simulink model "Tester"  (R2023b)
settings: Solver=VariableStepAuto  StartTime=0.0  StopTime=10.0  RelTol=1e-3
undefined symbols (not defined in the file or in its folder): canChannel
libraries: nesl_utility x9, fl_lib x8, ee_lib x6, canmsglib x3, canlib x2
settings Model: Creator=diego  LastModifiedBy=diego

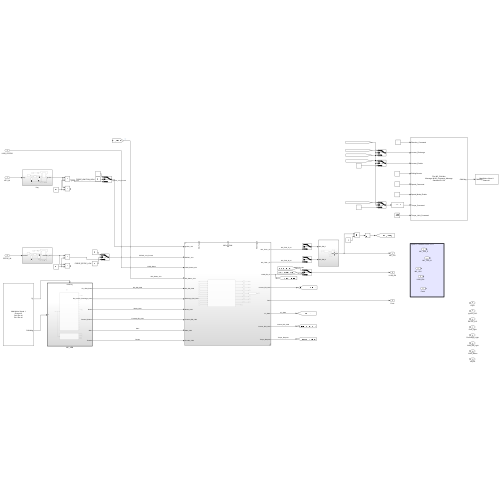
[thumbnail: Simulink's stored preview of the top-level diagram]
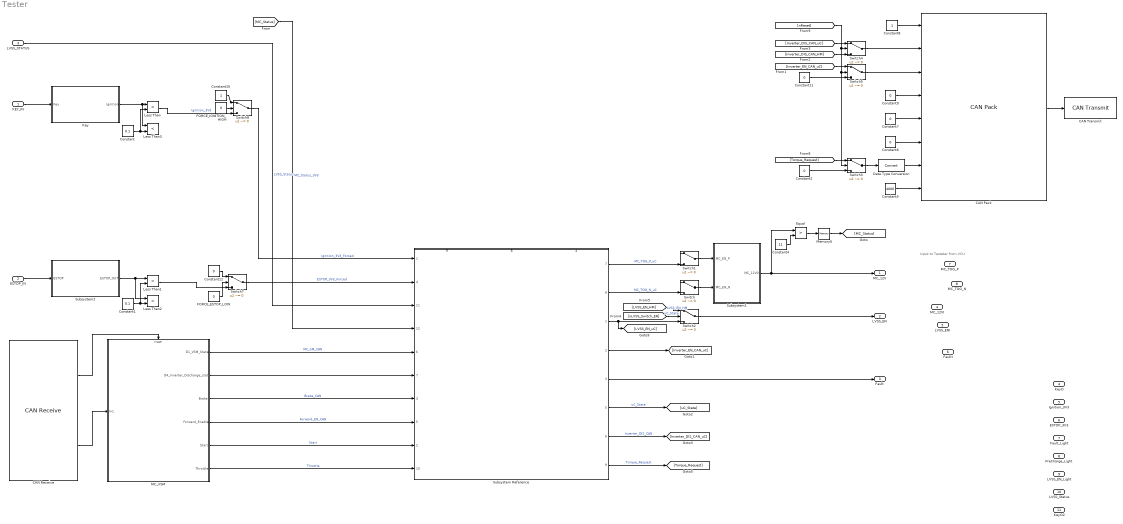
== system Tester ==
  note: Input to Testeter from VCU
  KEY_IN : Inport
  ESTOP_IN : Inport  Port=2
  LVSS_STATUS : Inport  Port=3  OutDataTypeStr=boolean
  MC_12VI : Inport  Port=4
  LVSS_ENI : Inport  Port=5
  FaultI : Inport  Port=6
  MC_TOG_P : Inport  Port=7
  MC_TOG_N : Inport  Port=8
  CAN Pack : canmsglib/CAN Pack  CANdbFile=C:\Users\heyka\MATLAB\Projects\VCU_C\MC_CAN.dbc  MsgList=M192_Command_Message  MsgName=M192_Command_Message  MsgIDType=Standard (11-bit identifier)  MsgIdentifier=192  MsgLength=8  Remote=off  ApplyMinMax=off  BusOutput=off  SignalInfo={'Direction_Command','32','1','LE','unsigned','Standard','0','1','0','0','1';'Inverter_Discharge','41','1','LE','unsigned','Standard','0','1','0','0','1';'Inverter_Enable','40','1','LE','unsigned','Standard','0','1','0','0','1';'RollingCounter','44','4','LE','unsigned','Standard','0','1','0','0','15';'Speed_Command','16','16','LE','signed','Standard','0','1','0','-32768','32767';'Speed_Mode_Enable','42','1','LE','unsigned','Standard','0','1','0','0','1';'Torque_Command','0','16','LE','signed','Standard','0','0.1','0','-3276.8','3276.7';'Torque_Limit_Command','48','16','LE','signed','Standard','0','0.1','0','-3276.8','3276.7'}
      settings: LibrarySourceBlock=canlib/CAN Pack  DataFormat=CANdb specified signals
  CAN Receive : canlib/CAN Receive  BlockHandle=405.006  Device=MathWorks Virtual 1 (Channel 2)  DeviceMenu=MathWorks Virtual 1 (Channel 2)  ObjConstructor=canChannel('MathWorks', 'Virtual 1', 2)  EnableStandardIDsFilter=off  StdIDsCombo=Allow all  StandardIDs=0  EnableExtendedIDsFilter=off  ExtIDsCombo=Allow all  ExtendedIDs=0  SampleTime=0.01  MsgsPerTimestep=all  InternalFilterUpdateStatus=on  BusOutput=off
  CAN Transmit : canlib/CAN Transmit  BlockHandle=406.006  Device=MathWorks Virtual 1 (Channel 1)  DeviceMenu=MathWorks Virtual 1 (Channel 1)  ObjConstructor=canChannel('MathWorks', 'Virtual 1', 1)  EnableEventTransmit=off  EnablePeriodicTransmit=off  MessagePeriod=1.000
  Constant : Constant  Value=0.1
  Constant1 : Constant  Value=0.1
  Constant10 : Constant  OutDataTypeStr=boolean
  Constant{2,6..7,9,11} (5 alike) : Constant  Value=0
  Constant12 : Constant  Value=0  OutDataTypeStr=boolean
  Constant4 : Constant  Value=11
  Constant5 : Constant  Value=4000
  Constant8 : Constant
  Data Type Conversion : DataTypeConversion  OutMin=[-32768]  OutMax=[32767]  SaturateOnIntegerOverflow=off  RndMeth=Floor
  Equal : RelationalOperator  Operator=>  OutDataTypeStr=boolean  RndMeth=Simplest  InputSameDT=off
  FORCE_ESTOP_LOW : Constant  Value=0
  FORCE_IGNITION_HIGH : Constant  Value=0
  Key : Subsystem
  Less Than{,1..3} (4 alike) : RelationalOperator  Operator=<  OutDataTypeStr=boolean  RndMeth=Simplest  InputSameDT=off
  MC_VSM : Subsystem  TreatAsAtomicUnit=on
  Memory6 : Memory
  Subsystem Reference : Subsystem  ReferencedSubsystem=MCuC_CAN
      settings: PortSchema="{\"entries\":[{\"content\":{\"sides\":[{\"content\":{\"connectorIds\":[\"In1\",\"In4\",\"In11\",\"In12\",\"In6\",\"In7\",\"In3\",\"In5\",\"In2\",\"In10\"]},\"type\":\"ConnectorPlacement.EquallySpacedRectSide\",\"uuid\":\"ad24675a-cf45-4ebd-8a91-6dc83f3b6f0e\"},{\"content\":{\"connectorIds\":[\"Out7\",\"Out8\",\"Out1\",\"Out2\",\"Out3\",\"Out5\",\"Out6\",\"Out9\"],\"side\":\"RIGHT\"},\"type\":\"ConnectorPlacement.EquallySpacedRectSide\",\"uuid\":\"d727ad1f-9d18-4e4b-88a0-ff4b62c4d504\"},{\"content\":{\"connectorIds\":[\"In9\",\"In8\",\"Out4\"],\"side\":\"TOP\"},\"type\":\"ConnectorPlacement.EquallySpacedRectSide\",\"uuid\":\"0dd4e640-1d3d-4994-a378-fd1340433361\"}]},\"type\":\"ConnectorPlacement.EquallySpacedConnector\",\"uuid\":\"60e23daf-f786-4411-86d8-86e23e1960b1\"}],\"packageUris\":[\"http://schema.mathworks.com/mf0/Connector/R2020b\"],\"version\":\"1.0\"}"
  Subsystem1 : Subsystem
  Subsystem2 : Subsystem
  Switch{,1..5} (6 alike) : Switch  Criteria=u2 ~= 0  SaturateOnIntegerOverflow=off  InputSameDT=off
  Switch7 : Switch  Criteria=u2 ~= 0  OutDataTypeStr=boolean  SaturateOnIntegerOverflow=off  InputSameDT=off
  Switch8 : Switch  Criteria=u2 ~= 0  OutDataTypeStr=boolean  SaturateOnIntegerOverflow=off  InputSameDT=off
  MC_12V : Outport
  LVSS_EN : Outport  Port=2
  Fault : Outport  Port=3
  KeyO : Outport  Port=4
  Ignition_3V3 : Outport  Port=5
  ESTOP_3V3 : Outport  Port=6
  Fault_Light : Outport  Port=7
  PreCharge_Light : Outport  Port=8
  LVSS_EN_Light : Outport  Port=9
  LVSS_Status : Outport  Port=10
  KeyO2 : Outport  Port=11
  wires:
  Subsystem Reference/2 -> [Inverter_EN_CAN_uC]
  Subsystem Reference/8 -> Switch/3  "MC_TOG_N_uC"
  Subsystem Reference/6 -> [Inverter_DIS_CAN_uC]  "Inverter_DIS_CAN"
  FORCE_ESTOP_LOW/1 -> Switch7/2
  Constant7/1 -> CAN Pack/5
  [Inverter_EN_CAN_uC] -> Switch5/1
  FORCE_IGNITION_HIGH/1 -> Switch8/2
  Less Than/1 -> Switch8/3  "Ignition_3V3"
  Constant10/1 -> Switch8/1
  LVSS_STATUS/1 -> Subsystem Reference/11  "LVSS_Status"
  Constant12/1 -> Switch7/1
  [Inverter_DIS_CAN_uC] -> Switch4/1
  KEY_IN/1 -> Key/1(Key)
  Subsystem Reference/9 -> [Torque_Request]  "Torque_Request"
  Switch1/1 -> Subsystem1/1(MC_EN_P)
  CAN Receive/1 -> MC_VSM/Trigger
  Switch7/1 -> Subsystem Reference/4  "ESTOP_3V3_Forced"
  Subsystem2/1(ESTOP_OUT) -> Less Than1/1, Less Than2/1
  [LVSS_EN_HM] -> Switch2/1  "LVSS_EN_HM"
  Constant2/1 -> Switch3/3
  Subsystem Reference/5 -> [uC_State]  "uC_State"
  MC_VSM/6(Throttle) -> Subsystem Reference/10  "Throttle"
  CAN Pack/1 -> CAN Transmit/1
  [MC_Status] -> Subsystem Reference/12  "MC_Status_3V3"
  CAN Receive/2 -> MC_VSM/1(In1)
  [nReset] -> Switch3/2, Switch5/2, Switch4/2
  ESTOP_IN/1 -> Subsystem2/1(ESTOP)
  MC_VSM/5(Start) -> Subsystem Reference/2  "Start"
  Subsystem Reference/7 -> Switch1/3  "MC_TOG_P_uC"
  [nLVSS_Switch_EN] -> Switch2/2  "uC_State"
  MC_VSM/2(D4_Inverter_Discharge_state) -> Subsystem Reference/7
  Switch8/1 -> Subsystem Reference/1  "Ignition_3V3_Forced"
  Subsystem Reference/1 -> [LVSS_EN_uC], Switch2/3
  Switch/1 -> Subsystem1/2(MC_EN_N)
  Constant1/1 -> Less Than1/2, Less Than2/2
  Constant11/1 -> Switch5/3
  Data Type Conversion/1 -> CAN Pack/7
  Constant6/1 -> CAN Pack/6
  Constant5/1 -> CAN Pack/8
  Equal/1 -> Memory6/1
  MC_VSM/1(D1_VSM_State) -> Subsystem Reference/6  "MC_SM_CAN"
  Constant4/1 -> Equal/2
  Key/1(Ignition) -> Less Than3/1, Less Than/1
  MC_VSM/4(Forward_Enable) -> Subsystem Reference/5  "Forward_EN_CAN"
  Switch2/1 -> LVSS_EN/1
  MC_VSM/3(Brake) -> Subsystem Reference/3  "Brake_CAN"
  [Inverter_DIS_CAN_HM] -> Switch4/3
  Switch3/1 -> Data Type Conversion/1
  Switch4/1 -> CAN Pack/2
  Constant/1 -> Less Than/2, Less Than3/2
  Subsystem1/1(MC_12V0) -> MC_12V/1, Equal/1
  Switch5/1 -> CAN Pack/3
  Less Than1/1 -> Switch7/3
  Subsystem Reference/3 -> Fault/1
  Constant8/1 -> CAN Pack/1
  Constant9/1 -> CAN Pack/4
  [Torque_Request] -> Switch3/1
  Memory6/1 -> [MC_Status]

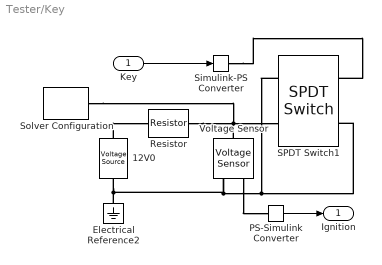
== system Tester/Key ==
  Key : Inport
  12V0 : ee_lib/Sources/Voltage Source  dc_voltage=12 V  ac_voltage=0 V  ac_shift=0 rad  ac_frequency=60 Hz  noise_mode=ee.enum.sources.noise.Disabled  PSD=0 V^2/Hz  sample_time=1e-3 s  repeatability=ee.enum.sources.repeatability.NotRepeatable  user_seed=0  auto_seed=3499211588  i_specify=off  i_priority=None  i=0 A  i_nominal_specify=off  i_nominal_unit=A  i_nominal_value=1  v_specify=off  v_priority=None  v=0 V  v_nominal_specify=off  v_nominal_unit=V  v_nominal_value=1
  Electrical Reference2 : fl_lib/Electrical/Electrical Elements/Electrical Reference
  PS-Simulink Converter : nesl_utility/PS-Simulink Converter  PhysicalDomain=network_engine_domain  SubClassName=ps_output  LeftPortType=input  RightPortType=output  PseudoPeriodic=off  Frequencies=[]  VectorFormat=inherit  Unit=inherit  AffineConversion=off
  Resistor : fl_lib/Electrical/Electrical Elements/Resistor  R=10000 Ohm  i_specify=off  i_priority=None  i=0 A  i_nominal_specify=off  i_nominal_unit=A  i_nominal_value=1  v_specify=off  v_priority=None  v=0 V  v_nominal_specify=off  v_nominal_unit=V  v_nominal_value=1
  SPDT Switch1 : ee_lib/Switches & Breakers/SPDT Switch  R_closed=0.01 Ohm  G_open=1e-10 S  Threshold=0.5 V  Width=0 V  model_dynamics=0  t_on=1e-3 s  t_off=1e-3 s  initial_vT=0 V
  Simulink-PS Converter : nesl_utility/Simulink-PS Converter  PhysicalDomain=network_engine_domain  SubClassName=ps_input  LeftPortType=input  RightPortType=output  PseudoPeriodic=off  Frequencies=[]  NoiseDistribution=none  NoiseParameters=[]  Unit=1  AffineConversion=off  FilteringAndDerivatives=provide  SimscapeFilterOrder=1  InputFilterTimeConstant=0.001  UdotUserProvided=0
  Solver Configuration : nesl_utility/Solver Configuration  PhysicalDomain=network_engine_domain  SubClassName=solver  LeftPortType=input  RightPortType=generic  Tones=[]  Harmonics=[]  SimulateNoise=off  Profile=off  UseLocalSampling=off  EnableSwitchedLinearOptims=on  FrequencyDomain=off  UseCCode=off  RelTol=0.001  AbsTol=0.001  MinStep=1e-09  ToWorkspace=off  RevertToSquareIcSolve=off  NumHomotopyIterations=100  PhasorMode=off  PhasorModeNumHarmonics=1  ConsistencySolver=NEWTON_XTOL_AFTER_FTOL  IndexReductionMethod=DerivativeReplacement  DoDC=off  ResidualTolerance=1e-09  ConsistencyTolSource=GLOBAL  ConsistencyAbsTol=0.001  ConsistencyRelTol=0.001  ConsistencyTolFactor=0.001  UseLocalSolver=off  LocalSolverChoice=NE_BACKWARD_EULER_ADVANCER  ResolveIndetEquations=on  FunctionEvalNumThread=1  LocalSolverSampleTime=0.001  DoFixedCost=off  MaxNonlinIter=3  MaxModeIter=2  ComputeImpulses=off  ImpulseIterations=2  LinearAlgebra=auto  LinearAlgebraNumThread=0  EquationFormulation=NE_TIME_EF  DelaysMemoryBudget=1024  AutomaticFiltering=on  FilteringTimeConstant=0.001  PartitionStorageMethod=AS_NEEDED  PartitionMemoryBudget=1024  PartitionMethod=ROBUST  MultibodyUseLocalSolver=off  MultibodyLocalSolverChoice=ODE1  MultibodyLocalSolverSampleTime=0.001
  Voltage Sensor : fl_lib/Electrical/Electrical Sensors/Voltage Sensor
  Ignition : Outport
  wires:
  PS-Simulink Converter/1 -> Ignition/1
  Key/1 -> Simulink-PS Converter/1
  connections:
  12V0/LConn1 -- Resistor/LConn1
  Resistor/RConn1 -- Solver Configuration/RConn1 -- Voltage Sensor/LConn1 -- SPDT Switch1/RConn2
  Electrical Reference2/LConn1 -- SPDT Switch1/RConn1 -- SPDT Switch1/LConn2 -- Voltage Sensor/RConn2 -- 12V0/RConn1
  Simulink-PS Converter/RConn1 -- SPDT Switch1/LConn1
  Voltage Sensor/RConn1 -- PS-Simulink Converter/LConn1

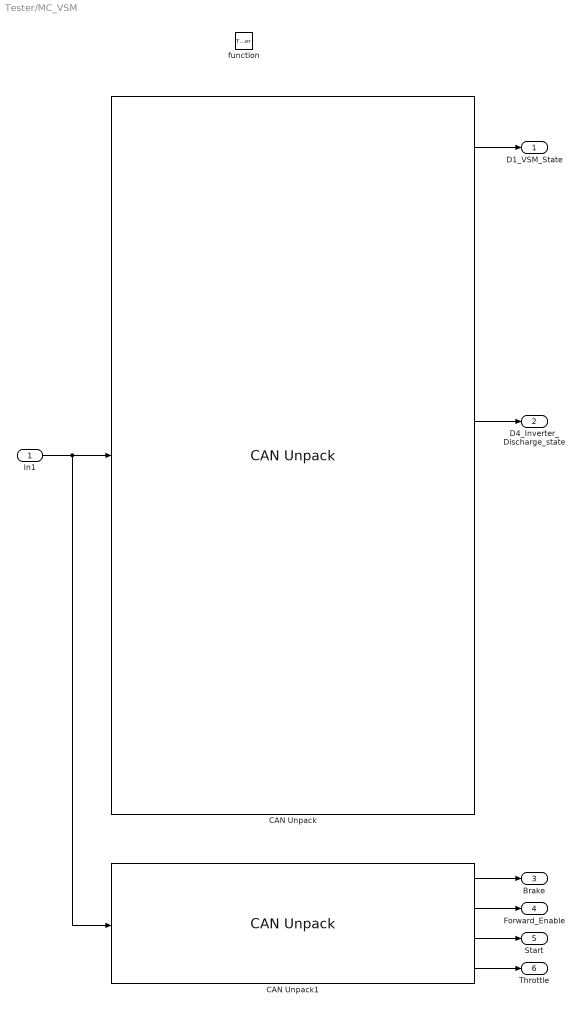
== system Tester/MC_VSM ==
  In1 : Inport
  function : TriggerPort  TriggerType=function-call  VariantControl=(inherit)
  CAN Unpack : canmsglib/CAN Unpack  CANdbFile=C:\Users\heyka\MATLAB\Projects\VCU_C\MC_CAN.dbc  MsgList=M170_Internal_States  MsgName=M170_Internal_States  MsgIDType=Standard (11-bit identifier)  MsgIdentifier=170  MsgLength=8  SignalInfo={'D1_PWM_Frequency','8','8','LE','unsigned','Standard','0','1','0','0','255';'D1_VSM_State','0','8','LE','unsigned','Standard','0','1','0','0','15';'D2_Inverter_State','16','8','LE','unsigned','Standard','0','1','0','0','255';'D3_Relay_1_Status','24','1','LE','unsigned','Standard','0','1','0','0','1';'D3_Relay_2_Status','25','1','LE','unsigned','Standard','0','1','0','0','1';'D3_Relay_3_Status','26','1','LE','unsigned','Standard','0','1','0','0','1';'D3_Relay_4_Status','27','1','LE','unsigned','Standard','0','1','0','0','1';'D3_Relay_5_Status','28','1','LE','unsigned','Standard','0','1','0','0','1';'D3_Relay_6_Status','29','1','LE','unsigned','Standard','0','1','0','0','1';'D4_Inverter_Discharge_State','37','3','LE','unsigned','Standard','0','1','0','0','7';'D4_Inverter_Run_Mode','32','1','LE','unsigned','Standard','0','1','0','0','1';'D5_Inverter_Command_Mode','40','1','LE','unsigned','Standard','0','1','0','0','1';'D5_Rolling_Counter','44','4','LE','unsigned','Standard','0','1','0','0','15';'D6_Inverter_Enable_Lockout','55','1','LE','unsigned','Standard','0','1','0','0','1';'D6_Inverter_Enable_State','48','1','LE','unsigned','Standard','0','1','0','0','1';'D6_Start_Mode_Active','54','1','LE','unsigned','Standard','0','1','0','0','1';'D7_BMS_Active','57','1','LE','unsigned','Standard','0','1','0','0','1';'D7_BMS_Torque_Limiting','58','1','LE','unsigned','Standard','0','1','0','0','1';'D7_Direction_Command','56','1','LE','unsigned','Standard','0','1','0','0','1';'D7_Low_Speed_Limiting','61','1','LE','unsigned','Standard','0','1','0','0','1';'D7_Max_Speed_Limiting','59','1','LE','unsigned','Standard','0','1','0','0','1'}  IDPort=off  TimestampPort=off  ErrorPort=off  RemotePort=off  LengthPort=off  StatusPort=off  ApplyMinMax=off
      settings: LibrarySourceBlock=canlib/CAN Unpack  DataFormat=CANdb specified signals
  CAN Unpack1 : canmsglib/CAN Unpack  CANdbFile=C:\Users\heyka\MATLAB\Projects\VCU_C\PRJDB.dbc  MsgList=N8_TPDO0  MsgName=N8_TPDO0  MsgIDType=Standard (11-bit identifier)  MsgIdentifier=392  MsgLength=5  SignalInfo={'Brake','1','16','LE','signed','Standard','0','1','0','0','494967295';'Forward_Enable','0','1','LE','unsigned','Standard','0','1','0','0','494967295';'Start','17','1','LE','unsigned','Standard','0','1','0','-Inf','Inf';'Throttle','18','16','LE','signed','Standard','0','1','0','-32768','32767'}  IDPort=off  TimestampPort=off  ErrorPort=off  RemotePort=off  LengthPort=off  StatusPort=off  ApplyMinMax=off
      settings: LibrarySourceBlock=canlib/CAN Unpack  DataFormat=CANdb specified signals
  D1_VSM_State : Outport
  D4_Inverter_Discharge_state : Outport  Port=2
  Brake : Outport  Port=3  OutDataTypeStr=int32
  Forward_Enable : Outport  Port=4  OutDataTypeStr=uint32
  Start : Outport  Port=5  OutDataTypeStr=uint32
  Throttle : Outport  Port=6  OutDataTypeStr=int32
  wires:
  In1/1 -> CAN Unpack1/1, CAN Unpack/1
  CAN Unpack/2 -> D1_VSM_State/1
  CAN Unpack/10 -> D4_Inverter_Discharge_state/1
  CAN Unpack1/1 -> Brake/1
  CAN Unpack1/2 -> Forward_Enable/1
  CAN Unpack1/3 -> Start/1
  CAN Unpack1/4 -> Throttle/1

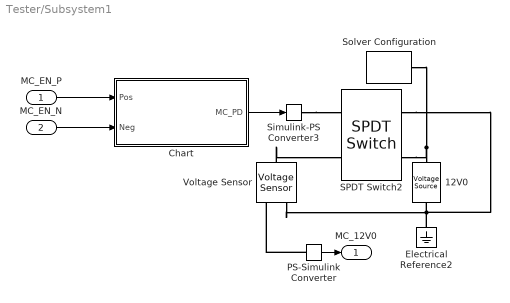
== system Tester/Subsystem1 ==
  MC_EN_P : Inport
  MC_EN_N : Inport  Port=2
  12V0 : ee_lib/Sources/Voltage Source  dc_voltage=12 V  ac_voltage=0 V  ac_shift=0 rad  ac_frequency=60 Hz  noise_mode=ee.enum.sources.noise.Disabled  PSD=0 V^2/Hz  sample_time=1e-3 s  repeatability=ee.enum.sources.repeatability.NotRepeatable  user_seed=0  auto_seed=3890346746  i_specify=off  i_priority=None  i=0 A  i_nominal_specify=off  i_nominal_unit=A  i_nominal_value=1  v_specify=off  v_priority=None  v=0 V  v_nominal_specify=off  v_nominal_unit=V  v_nominal_value=1
  Chart : Stateflow chart  TreatAsAtomicUnit=on
  Electrical Reference2 : fl_lib/Electrical/Electrical Elements/Electrical Reference
  PS-Simulink Converter : nesl_utility/PS-Simulink Converter  PhysicalDomain=network_engine_domain  SubClassName=ps_output  LeftPortType=input  RightPortType=output  PseudoPeriodic=off  Frequencies=[]  VectorFormat=inherit  Unit=inherit  AffineConversion=off
  SPDT Switch2 : ee_lib/Switches & Breakers/SPDT Switch  R_closed=0.01 Ohm  G_open=1e-6 S  Threshold=0.5 V  Width=0 V  model_dynamics=0  t_on=1e-3 s  t_off=1e-3 s  initial_vT=0 V
  Simulink-PS Converter3 : nesl_utility/Simulink-PS Converter  PhysicalDomain=network_engine_domain  SubClassName=ps_input  LeftPortType=input  RightPortType=output  PseudoPeriodic=off  Frequencies=[]  NoiseDistribution=none  NoiseParameters=[]  Unit=1  AffineConversion=off  FilteringAndDerivatives=provide  SimscapeFilterOrder=1  InputFilterTimeConstant=0.001  UdotUserProvided=0
  Solver Configuration : nesl_utility/Solver Configuration  PhysicalDomain=network_engine_domain  SubClassName=solver  LeftPortType=input  RightPortType=generic  Tones=[]  Harmonics=[]  SimulateNoise=off  Profile=off  UseLocalSampling=off  EnableSwitchedLinearOptims=on  FrequencyDomain=off  UseCCode=off  RelTol=0.001  AbsTol=0.001  MinStep=1e-09  ToWorkspace=off  RevertToSquareIcSolve=off  NumHomotopyIterations=100  PhasorMode=off  PhasorModeNumHarmonics=1  ConsistencySolver=NEWTON_XTOL_AFTER_FTOL  IndexReductionMethod=DerivativeReplacement  DoDC=off  ResidualTolerance=1e-09  ConsistencyTolSource=GLOBAL  ConsistencyAbsTol=0.001  ConsistencyRelTol=0.001  ConsistencyTolFactor=0.001  UseLocalSolver=off  LocalSolverChoice=NE_BACKWARD_EULER_ADVANCER  ResolveIndetEquations=on  FunctionEvalNumThread=1  LocalSolverSampleTime=0.001  DoFixedCost=off  MaxNonlinIter=3  MaxModeIter=2  ComputeImpulses=off  ImpulseIterations=2  LinearAlgebra=auto  LinearAlgebraNumThread=0  EquationFormulation=NE_TIME_EF  DelaysMemoryBudget=1024  AutomaticFiltering=on  FilteringTimeConstant=0.001  PartitionStorageMethod=AS_NEEDED  PartitionMemoryBudget=1024  PartitionMethod=ROBUST  MultibodyUseLocalSolver=off  MultibodyLocalSolverChoice=ODE1  MultibodyLocalSolverSampleTime=0.001
  Voltage Sensor : fl_lib/Electrical/Electrical Sensors/Voltage Sensor
  MC_12V0 : Outport
  wires:
  MC_EN_P/1 -> Chart/1(Pos)
  MC_EN_N/1 -> Chart/2(Neg)
  Chart/1(MC_PD) -> Simulink-PS Converter3/1
  PS-Simulink Converter/1 -> MC_12V0/1
  connections:
  Simulink-PS Converter3/RConn1 -- SPDT Switch2/LConn1
  PS-Simulink Converter/LConn1 -- Voltage Sensor/RConn1
  Electrical Reference2/LConn1 -- 12V0/RConn1 -- Voltage Sensor/RConn2 -- SPDT Switch2/RConn1
  SPDT Switch2/RConn2 -- Solver Configuration/RConn1 -- 12V0/LConn1
  Voltage Sensor/LConn1 -- SPDT Switch2/LConn2

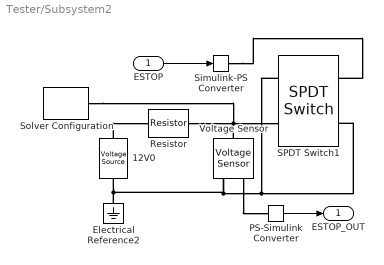
== system Tester/Subsystem2 ==
  ESTOP : Inport
  12V0 : ee_lib/Sources/Voltage Source  dc_voltage=12 V  ac_voltage=0 V  ac_shift=0 rad  ac_frequency=60 Hz  noise_mode=ee.enum.sources.noise.Disabled  PSD=0 V^2/Hz  sample_time=1e-3 s  repeatability=ee.enum.sources.repeatability.NotRepeatable  user_seed=0  auto_seed=545404223  i_specify=off  i_priority=None  i=0 A  i_nominal_specify=off  i_nominal_unit=A  i_nominal_value=1  v_specify=off  v_priority=None  v=0 V  v_nominal_specify=off  v_nominal_unit=V  v_nominal_value=1
  Electrical Reference2 : fl_lib/Electrical/Electrical Elements/Electrical Reference
  PS-Simulink Converter : nesl_utility/PS-Simulink Converter  PhysicalDomain=network_engine_domain  SubClassName=ps_output  LeftPortType=input  RightPortType=output  PseudoPeriodic=off  Frequencies=[]  VectorFormat=inherit  Unit=inherit  AffineConversion=off
  Resistor : fl_lib/Electrical/Electrical Elements/Resistor  R=10000 Ohm  i_specify=off  i_priority=None  i=0 A  i_nominal_specify=off  i_nominal_unit=A  i_nominal_value=1  v_specify=off  v_priority=None  v=0 V  v_nominal_specify=off  v_nominal_unit=V  v_nominal_value=1
  SPDT Switch1 : ee_lib/Switches & Breakers/SPDT Switch  R_closed=0.01 Ohm  G_open=1e-10 S  Threshold=0.5 V  Width=0 V  model_dynamics=0  t_on=1e-3 s  t_off=1e-3 s  initial_vT=0 V
  Simulink-PS Converter : nesl_utility/Simulink-PS Converter  PhysicalDomain=network_engine_domain  SubClassName=ps_input  LeftPortType=input  RightPortType=output  PseudoPeriodic=off  Frequencies=[]  NoiseDistribution=none  NoiseParameters=[]  Unit=1  AffineConversion=off  FilteringAndDerivatives=provide  SimscapeFilterOrder=1  InputFilterTimeConstant=0.001  UdotUserProvided=0
  Solver Configuration : nesl_utility/Solver Configuration  PhysicalDomain=network_engine_domain  SubClassName=solver  LeftPortType=input  RightPortType=generic  Tones=[]  Harmonics=[]  SimulateNoise=off  Profile=off  UseLocalSampling=off  EnableSwitchedLinearOptims=on  FrequencyDomain=off  UseCCode=off  RelTol=0.001  AbsTol=0.001  MinStep=1e-09  ToWorkspace=off  RevertToSquareIcSolve=off  NumHomotopyIterations=100  PhasorMode=off  PhasorModeNumHarmonics=1  ConsistencySolver=NEWTON_XTOL_AFTER_FTOL  IndexReductionMethod=DerivativeReplacement  DoDC=off  ResidualTolerance=1e-09  ConsistencyTolSource=GLOBAL  ConsistencyAbsTol=0.001  ConsistencyRelTol=0.001  ConsistencyTolFactor=0.001  UseLocalSolver=off  LocalSolverChoice=NE_BACKWARD_EULER_ADVANCER  ResolveIndetEquations=on  FunctionEvalNumThread=1  LocalSolverSampleTime=0.001  DoFixedCost=off  MaxNonlinIter=3  MaxModeIter=2  ComputeImpulses=off  ImpulseIterations=2  LinearAlgebra=auto  LinearAlgebraNumThread=0  EquationFormulation=NE_TIME_EF  DelaysMemoryBudget=1024  AutomaticFiltering=on  FilteringTimeConstant=0.001  PartitionStorageMethod=AS_NEEDED  PartitionMemoryBudget=1024  PartitionMethod=ROBUST  MultibodyUseLocalSolver=off  MultibodyLocalSolverChoice=ODE1  MultibodyLocalSolverSampleTime=0.001
  Voltage Sensor : fl_lib/Electrical/Electrical Sensors/Voltage Sensor
  ESTOP_OUT : Outport
  wires:
  PS-Simulink Converter/1 -> ESTOP_OUT/1
  ESTOP/1 -> Simulink-PS Converter/1
  connections:
  12V0/LConn1 -- Resistor/LConn1
  Voltage Sensor/LConn1 -- SPDT Switch1/RConn2 -- Resistor/RConn1 -- Solver Configuration/RConn1
  SPDT Switch1/LConn2 -- 12V0/RConn1 -- Electrical Reference2/LConn1 -- Voltage Sensor/RConn2 -- SPDT Switch1/RConn1
  Simulink-PS Converter/RConn1 -- SPDT Switch1/LConn1
  Voltage Sensor/RConn1 -- PS-Simulink Converter/LConn1

== stateflow chart Tester/Subsystem1/Chart ==
  state Relay_Open
    MC_PD = 0;
  state Relay_Close
    MC_PD = 1;
  (default) -> Relay_Open
  Relay_Open -> Relay_Close : [Pos == 1 && Neg == 0]
  Relay_Close -> Relay_Open : [Pos == 0 && Neg == 1]
  data: Pos input; MC_PD output =0; Neg input
